simulink model "bb_test"  (R2013b)
settings: Solver=ode45  StartTime=0.0  StopTime=10.0  RelTol=1e-3
libraries: xbsIndex_r4 x4
settings Model: Creator=root  LastModifiedBy=root

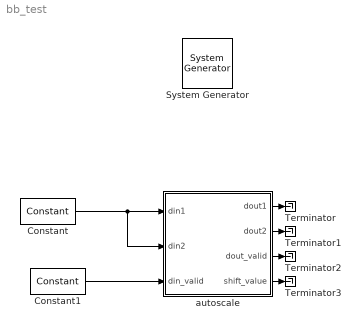
== system bb_test ==
  " System Generator" : xbsIndex_r4/ System Generator  Tag=genX  xilinxfamily=Kintex7  part=xc7k325t  speed=-3  package=fbg676  synthesis_tool=XST  clock_wrapper=Clock Enables  directory=./netlist  proj_type=Project Navigator  Synth_file=XST Defaults  Impl_file=ISE Defaults  testbench=off  simulink_period=1  sysclk_period=10  dcm_input_clock_period=10  incr_netlist=off  trim_vbits=Everywhere in SubSystem  dbl_ovrd=According to Block Masks  core_generation=According to Block Masks  run_coregen=off  deprecated_control=off  eval_field=0  block_type=sysgen
  Constant : xbsIndex_r4/Constant  const=1  gui_display_data_type=Fixed-point  arith_type=Unsigned  n_bits=16  bin_pt=0  preci_type=Single  exp_width=8  frac_width=24  explicit_period=on  period=1  equ=P=C  opselect=C  inp2=PCIN>>17  opr=+  inp1=P  carry=CIN  dbl_ovrd=off  block_type=constant
  Constant1 : xbsIndex_r4/Constant  const=1  gui_display_data_type=Boolean  arith_type=Boolean  n_bits=16  bin_pt=0  preci_type=Single  exp_width=8  frac_width=24  explicit_period=on  period=1  equ=P=C  opselect=C  inp2=PCIN>>17  opr=+  inp1=P  carry=CIN  dbl_ovrd=off  block_type=constant
  Terminator{,1..3} (4 alike) : Terminator
  autoscale : Subsystem  mask{max_shift=10, min_shift=3, din_width=16}
      mask prompts: max_shift "max shift"; min_shift "min shift"; din_width "din width"
  wires:
  Constant/1 -> autoscale/2(din2), autoscale/1(din1)
  Constant1/1 -> autoscale/3(din_valid)
  autoscale/1(dout1) -> Terminator/1
  autoscale/2(dout2) -> Terminator1/1
  autoscale/3(dout_valid) -> Terminator2/1
  autoscale/4(shift_value) -> Terminator3/1

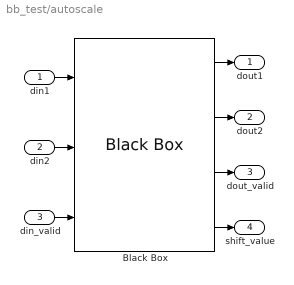
== system bb_test/autoscale ==
  din1 : Inport
  din2 : Inport  Port=2
  din_valid : Inport  Port=3
  Black Box : xbsIndex_r4/Black Box  init_code=autoscale_config  sim_method=Inactive  verbose=off  block_type=blackbox2
  dout1 : Outport
  dout2 : Outport  Port=2
  dout_valid : Outport  Port=3
  shift_value : Outport  Port=4
  wires:
  Black Box/3 -> dout_valid/1
  Black Box/4 -> shift_value/1
  din_valid/1 -> Black Box/3
  Black Box/2 -> dout2/1
  din1/1 -> Black Box/1
  din2/1 -> Black Box/2
  Black Box/1 -> dout1/1
